simulink model "RECEIVE_TEST"  (R2021b)
settings: Solver=VariableStepAuto  StartTime=0.0  StopTime=inf  RelTol=1e-3
undefined symbols (not defined in the file): f
libraries: instrumentlib x4
settings Model: Creator=ccortes9  LastModifiedBy=ccortes9

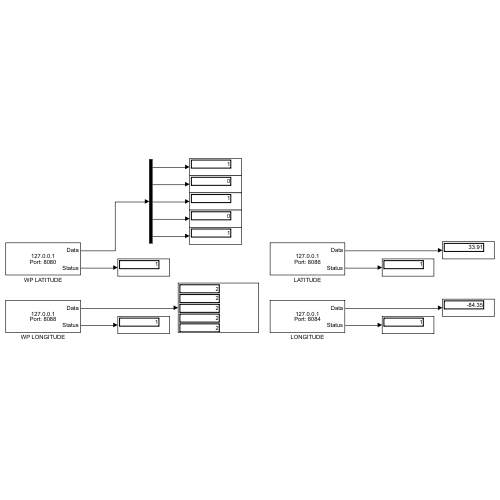
[thumbnail: Simulink's stored preview of the top-level diagram]
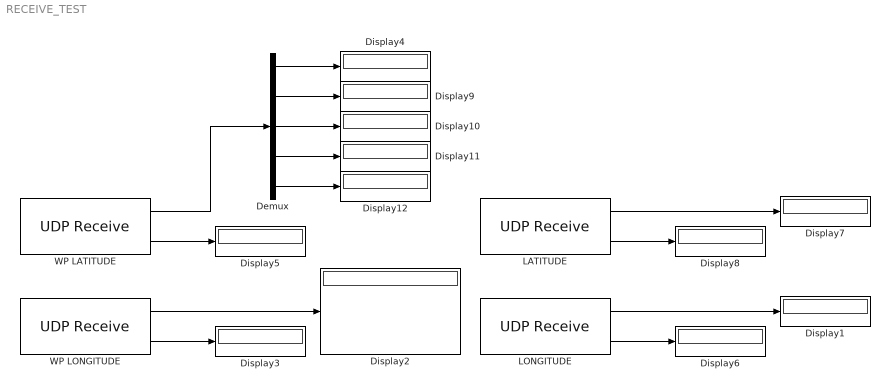
== system RECEIVE_TEST ==
  Demux : Demux  Outputs=5
  Display{1..12} (12 alike) : Display
  LATITUDE : instrumentlib/UDP Receive  Host=127.0.0.1  Port=8081  LocalPort=8086  EnablePortSharing=off  GetLatestData=off  DataSize=[1 1]  DataType=double  ASCIIFormatting=%f,  Terminator=LF  ByteOrder=BigEndian  EnableBlockingMode=off  Timeout=10  SampleTime=0.01  LocalAddress=127.0.0.1
  LONGITUDE : instrumentlib/UDP Receive  Host=127.0.0.1  Port=8083  LocalPort=8084  EnablePortSharing=off  GetLatestData=off  DataSize=[1 1]  DataType=double  ASCIIFormatting=%f,  Terminator=LF  ByteOrder=BigEndian  EnableBlockingMode=off  Timeout=10  SampleTime=0.01  LocalAddress=127.0.0.1
  WP LATITUDE : instrumentlib/UDP Receive  Host=127.0.0.1  Port=8087  LocalPort=8080  EnablePortSharing=off  GetLatestData=off  DataSize="[5  1]"  DataType=double  ASCIIFormatting=%f,  Terminator=LF  ByteOrder=BigEndian  EnableBlockingMode=off  Timeout=10  SampleTime=0.01  LocalAddress=127.0.0.1
  WP LONGITUDE : instrumentlib/UDP Receive  Host=127.0.0.1  Port=8089  LocalPort=8088  EnablePortSharing=off  GetLatestData=off  DataSize="[5  1]"  DataType=double  ASCIIFormatting=%f,  Terminator=LF  ByteOrder=BigEndian  EnableBlockingMode=off  Timeout=10  SampleTime=0.01  LocalAddress=127.0.0.1
  wires:
  WP LONGITUDE/1 -> Display2/1
  WP LATITUDE/2 -> Display5/1
  WP LONGITUDE/2 -> Display3/1
  LATITUDE/1 -> Display7/1
  LONGITUDE/2 -> Display6/1
  LONGITUDE/1 -> Display1/1
  LATITUDE/2 -> Display8/1
  WP LATITUDE/1 -> Demux/1
  Demux/2 -> Display9/1
  Demux/1 -> Display4/1
  Demux/3 -> Display10/1
  Demux/4 -> Display11/1
  Demux/5 -> Display12/1
